simulink model "gm_gmStateSpaceHDL_uz_inverter_3ph"  (R2021b)
settings: Solver=FixedStepDiscrete  StartTime=0.0  StopTime=0.1  FixedStep=Auto  RelTol=1e-3
InitFcn:
  | load('C:\Users\valen\Documents\repos\UZ\ultrazohm_sw_working\ip_cores\uz_inverter_3ph\sschdl\uz_inverter_3ph\stateSpaceParameters.mat');
undefined symbols (not defined in the file or in its folder): udc
libraries: hdlmdlgenlib x140, dspsigops x26, simulink x17, hdlssclib x2
(part 2 of 2)

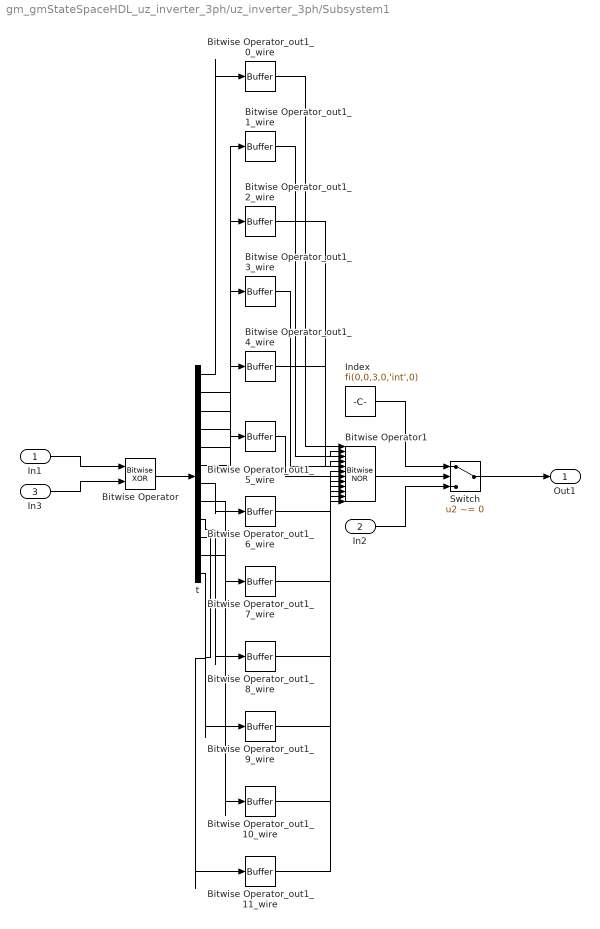
== system gm_gmStateSpaceHDL_uz_inverter_3ph/uz_inverter_3ph/Subsystem1 ==
  In1 : Inport  OutDataTypeStr=boolean  PortDimensions=[12]  SampleTime=1e-08
  In2 : Inport  Port=2  OutDataTypeStr=fixdt(0, 3, 0)  PortDimensions=1  SampleTime=1e-08
  In3 : Inport  Port=3  OutDataTypeStr=boolean  PortDimensions=[12]  SampleTime=1e-08
  Bitwise Operator : simulink/Logic and Bit Operations/Bitwise Operator  logicop=XOR  UseBitMask=off  NumInputPorts=2  BitMask=double(0)  BitMaskRealWorld=Real World Value
  Bitwise Operator1 : simulink/Logic and Bit Operations/Bitwise Operator  logicop=NOR  UseBitMask=off  NumInputPorts=12  BitMask=double(0)  BitMaskRealWorld=Real World Value
  Bitwise Operator_out1_0_wire : hdlmdlgenlib/Buffer
      settings: SourceProductBaseCode=SL
  Bitwise Operator_out1_10_wire : hdlmdlgenlib/Buffer
      settings: SourceProductBaseCode=SL
  Bitwise Operator_out1_11_wire : hdlmdlgenlib/Buffer
      settings: SourceProductBaseCode=SL
  Bitwise Operator_out1_1_wire : hdlmdlgenlib/Buffer
      settings: SourceProductBaseCode=SL
  Bitwise Operator_out1_2_wire : hdlmdlgenlib/Buffer
      settings: SourceProductBaseCode=SL
  Bitwise Operator_out1_3_wire : hdlmdlgenlib/Buffer
      settings: SourceProductBaseCode=SL
  Bitwise Operator_out1_4_wire : hdlmdlgenlib/Buffer
      settings: SourceProductBaseCode=SL
  Bitwise Operator_out1_5_wire : hdlmdlgenlib/Buffer
      settings: SourceProductBaseCode=SL
  Bitwise Operator_out1_6_wire : hdlmdlgenlib/Buffer
      settings: SourceProductBaseCode=SL
  Bitwise Operator_out1_7_wire : hdlmdlgenlib/Buffer
      settings: SourceProductBaseCode=SL
  Bitwise Operator_out1_8_wire : hdlmdlgenlib/Buffer
      settings: SourceProductBaseCode=SL
  Bitwise Operator_out1_9_wire : hdlmdlgenlib/Buffer
      settings: SourceProductBaseCode=SL
  Index : Constant  Value=fi(0,0,3,0,'int',0)  OutDataTypeStr=fixdt(0, 3, 0)  SampleTime=1e-08
  Switch : Switch  Criteria=u2 ~= 0  Threshold=double(0)  OutDataTypeStr=fixdt(0, 3, 0)  SampleTime=1e-08
  t : Demux  Outputs=12
  Out1 : Outport  SampleTime=1e-08  VectorParamsAs1DForOutWhenUnconnected=off
  wires:
  Bitwise Operator/1 -> t/1
  Bitwise Operator1/1 -> Switch/2
  Bitwise Operator_out1_0_wire/1 -> Bitwise Operator1/1
  Bitwise Operator_out1_1_wire/1 -> Bitwise Operator1/2
  Bitwise Operator_out1_2_wire/1 -> Bitwise Operator1/3
  Bitwise Operator_out1_3_wire/1 -> Bitwise Operator1/4
  Bitwise Operator_out1_4_wire/1 -> Bitwise Operator1/5
  Bitwise Operator_out1_5_wire/1 -> Bitwise Operator1/6
  Bitwise Operator_out1_6_wire/1 -> Bitwise Operator1/7
  Bitwise Operator_out1_7_wire/1 -> Bitwise Operator1/8
  Bitwise Operator_out1_8_wire/1 -> Bitwise Operator1/9
  Bitwise Operator_out1_9_wire/1 -> Bitwise Operator1/10
  Bitwise Operator_out1_10_wire/1 -> Bitwise Operator1/11
  Bitwise Operator_out1_11_wire/1 -> Bitwise Operator1/12
  Index/1 -> Switch/1
  Switch/1 -> Out1/1
  t/1 -> Bitwise Operator_out1_0_wire/1
  t/2 -> Bitwise Operator_out1_1_wire/1
  t/3 -> Bitwise Operator_out1_2_wire/1
  t/4 -> Bitwise Operator_out1_3_wire/1
  t/5 -> Bitwise Operator_out1_4_wire/1
  t/6 -> Bitwise Operator_out1_5_wire/1
  t/7 -> Bitwise Operator_out1_6_wire/1
  t/8 -> Bitwise Operator_out1_7_wire/1
  t/9 -> Bitwise Operator_out1_8_wire/1
  t/10 -> Bitwise Operator_out1_9_wire/1
  t/11 -> Bitwise Operator_out1_10_wire/1
  t/12 -> Bitwise Operator_out1_11_wire/1
  In1/1 -> Bitwise Operator/1
  In2/1 -> Switch/3
  In3/1 -> Bitwise Operator/2

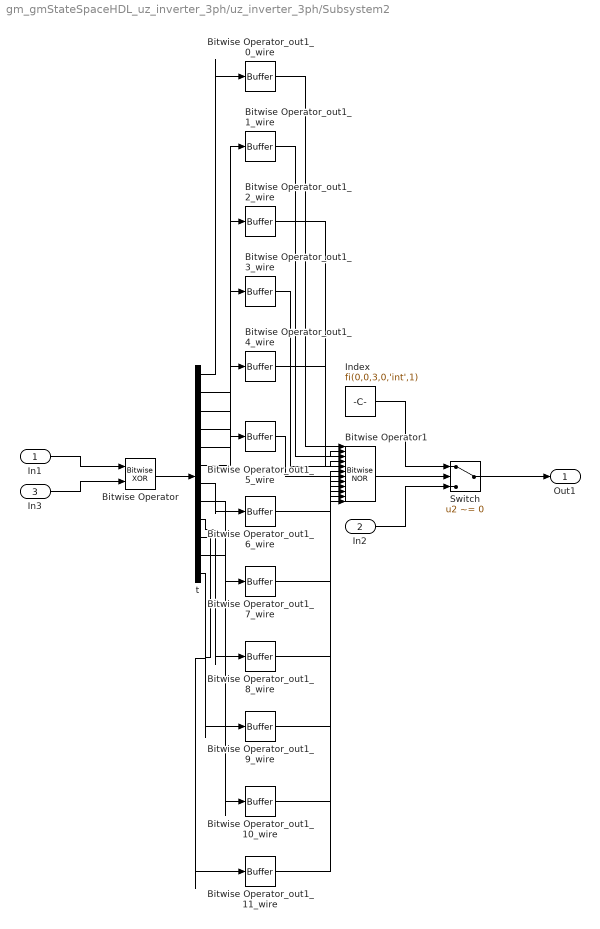
== system gm_gmStateSpaceHDL_uz_inverter_3ph/uz_inverter_3ph/Subsystem2 ==
  In1 : Inport  OutDataTypeStr=boolean  PortDimensions=[12]  SampleTime=1e-08
  In2 : Inport  Port=2  OutDataTypeStr=fixdt(0, 3, 0)  PortDimensions=1  SampleTime=1e-08
  In3 : Inport  Port=3  OutDataTypeStr=boolean  PortDimensions=[12]  SampleTime=1e-08
  Bitwise Operator : simulink/Logic and Bit Operations/Bitwise Operator  logicop=XOR  UseBitMask=off  NumInputPorts=2  BitMask=double(0)  BitMaskRealWorld=Real World Value
  Bitwise Operator1 : simulink/Logic and Bit Operations/Bitwise Operator  logicop=NOR  UseBitMask=off  NumInputPorts=12  BitMask=double(0)  BitMaskRealWorld=Real World Value
  Bitwise Operator_out1_0_wire : hdlmdlgenlib/Buffer
      settings: SourceProductBaseCode=SL
  Bitwise Operator_out1_10_wire : hdlmdlgenlib/Buffer
      settings: SourceProductBaseCode=SL
  Bitwise Operator_out1_11_wire : hdlmdlgenlib/Buffer
      settings: SourceProductBaseCode=SL
  Bitwise Operator_out1_1_wire : hdlmdlgenlib/Buffer
      settings: SourceProductBaseCode=SL
  Bitwise Operator_out1_2_wire : hdlmdlgenlib/Buffer
      settings: SourceProductBaseCode=SL
  Bitwise Operator_out1_3_wire : hdlmdlgenlib/Buffer
      settings: SourceProductBaseCode=SL
  Bitwise Operator_out1_4_wire : hdlmdlgenlib/Buffer
      settings: SourceProductBaseCode=SL
  Bitwise Operator_out1_5_wire : hdlmdlgenlib/Buffer
      settings: SourceProductBaseCode=SL
  Bitwise Operator_out1_6_wire : hdlmdlgenlib/Buffer
      settings: SourceProductBaseCode=SL
  Bitwise Operator_out1_7_wire : hdlmdlgenlib/Buffer
      settings: SourceProductBaseCode=SL
  Bitwise Operator_out1_8_wire : hdlmdlgenlib/Buffer
      settings: SourceProductBaseCode=SL
  Bitwise Operator_out1_9_wire : hdlmdlgenlib/Buffer
      settings: SourceProductBaseCode=SL
  Index : Constant  Value=fi(0,0,3,0,'int',1)  OutDataTypeStr=fixdt(0, 3, 0)  SampleTime=1e-08
  Switch : Switch  Criteria=u2 ~= 0  Threshold=double(0)  OutDataTypeStr=fixdt(0, 3, 0)  SampleTime=1e-08
  t : Demux  Outputs=12
  Out1 : Outport  SampleTime=1e-08  VectorParamsAs1DForOutWhenUnconnected=off
  wires:
  Bitwise Operator/1 -> t/1
  Bitwise Operator1/1 -> Switch/2
  Bitwise Operator_out1_0_wire/1 -> Bitwise Operator1/1
  Bitwise Operator_out1_1_wire/1 -> Bitwise Operator1/2
  Bitwise Operator_out1_2_wire/1 -> Bitwise Operator1/3
  Bitwise Operator_out1_3_wire/1 -> Bitwise Operator1/4
  Bitwise Operator_out1_4_wire/1 -> Bitwise Operator1/5
  Bitwise Operator_out1_5_wire/1 -> Bitwise Operator1/6
  Bitwise Operator_out1_6_wire/1 -> Bitwise Operator1/7
  Bitwise Operator_out1_7_wire/1 -> Bitwise Operator1/8
  Bitwise Operator_out1_8_wire/1 -> Bitwise Operator1/9
  Bitwise Operator_out1_9_wire/1 -> Bitwise Operator1/10
  Bitwise Operator_out1_10_wire/1 -> Bitwise Operator1/11
  Bitwise Operator_out1_11_wire/1 -> Bitwise Operator1/12
  Index/1 -> Switch/1
  Switch/1 -> Out1/1
  t/1 -> Bitwise Operator_out1_0_wire/1
  t/2 -> Bitwise Operator_out1_1_wire/1
  t/3 -> Bitwise Operator_out1_2_wire/1
  t/4 -> Bitwise Operator_out1_3_wire/1
  t/5 -> Bitwise Operator_out1_4_wire/1
  t/6 -> Bitwise Operator_out1_5_wire/1
  t/7 -> Bitwise Operator_out1_6_wire/1
  t/8 -> Bitwise Operator_out1_7_wire/1
  t/9 -> Bitwise Operator_out1_8_wire/1
  t/10 -> Bitwise Operator_out1_9_wire/1
  t/11 -> Bitwise Operator_out1_10_wire/1
  t/12 -> Bitwise Operator_out1_11_wire/1
  In1/1 -> Bitwise Operator/1
  In2/1 -> Switch/3
  In3/1 -> Bitwise Operator/2

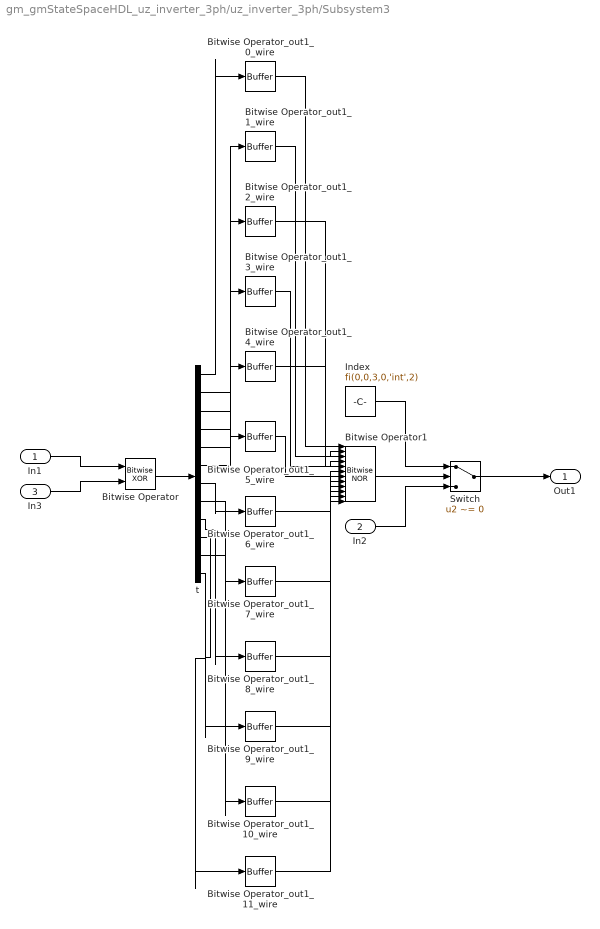
== system gm_gmStateSpaceHDL_uz_inverter_3ph/uz_inverter_3ph/Subsystem3 ==
  In1 : Inport  OutDataTypeStr=boolean  PortDimensions=[12]  SampleTime=1e-08
  In2 : Inport  Port=2  OutDataTypeStr=fixdt(0, 3, 0)  PortDimensions=1  SampleTime=1e-08
  In3 : Inport  Port=3  OutDataTypeStr=boolean  PortDimensions=[12]  SampleTime=1e-08
  Bitwise Operator : simulink/Logic and Bit Operations/Bitwise Operator  logicop=XOR  UseBitMask=off  NumInputPorts=2  BitMask=double(0)  BitMaskRealWorld=Real World Value
  Bitwise Operator1 : simulink/Logic and Bit Operations/Bitwise Operator  logicop=NOR  UseBitMask=off  NumInputPorts=12  BitMask=double(0)  BitMaskRealWorld=Real World Value
  Bitwise Operator_out1_0_wire : hdlmdlgenlib/Buffer
      settings: SourceProductBaseCode=SL
  Bitwise Operator_out1_10_wire : hdlmdlgenlib/Buffer
      settings: SourceProductBaseCode=SL
  Bitwise Operator_out1_11_wire : hdlmdlgenlib/Buffer
      settings: SourceProductBaseCode=SL
  Bitwise Operator_out1_1_wire : hdlmdlgenlib/Buffer
      settings: SourceProductBaseCode=SL
  Bitwise Operator_out1_2_wire : hdlmdlgenlib/Buffer
      settings: SourceProductBaseCode=SL
  Bitwise Operator_out1_3_wire : hdlmdlgenlib/Buffer
      settings: SourceProductBaseCode=SL
  Bitwise Operator_out1_4_wire : hdlmdlgenlib/Buffer
      settings: SourceProductBaseCode=SL
  Bitwise Operator_out1_5_wire : hdlmdlgenlib/Buffer
      settings: SourceProductBaseCode=SL
  Bitwise Operator_out1_6_wire : hdlmdlgenlib/Buffer
      settings: SourceProductBaseCode=SL
  Bitwise Operator_out1_7_wire : hdlmdlgenlib/Buffer
      settings: SourceProductBaseCode=SL
  Bitwise Operator_out1_8_wire : hdlmdlgenlib/Buffer
      settings: SourceProductBaseCode=SL
  Bitwise Operator_out1_9_wire : hdlmdlgenlib/Buffer
      settings: SourceProductBaseCode=SL
  Index : Constant  Value=fi(0,0,3,0,'int',2)  OutDataTypeStr=fixdt(0, 3, 0)  SampleTime=1e-08
  Switch : Switch  Criteria=u2 ~= 0  Threshold=double(0)  OutDataTypeStr=fixdt(0, 3, 0)  SampleTime=1e-08
  t : Demux  Outputs=12
  Out1 : Outport  SampleTime=1e-08  VectorParamsAs1DForOutWhenUnconnected=off
  wires:
  Bitwise Operator/1 -> t/1
  Bitwise Operator1/1 -> Switch/2
  Bitwise Operator_out1_0_wire/1 -> Bitwise Operator1/1
  Bitwise Operator_out1_1_wire/1 -> Bitwise Operator1/2
  Bitwise Operator_out1_2_wire/1 -> Bitwise Operator1/3
  Bitwise Operator_out1_3_wire/1 -> Bitwise Operator1/4
  Bitwise Operator_out1_4_wire/1 -> Bitwise Operator1/5
  Bitwise Operator_out1_5_wire/1 -> Bitwise Operator1/6
  Bitwise Operator_out1_6_wire/1 -> Bitwise Operator1/7
  Bitwise Operator_out1_7_wire/1 -> Bitwise Operator1/8
  Bitwise Operator_out1_8_wire/1 -> Bitwise Operator1/9
  Bitwise Operator_out1_9_wire/1 -> Bitwise Operator1/10
  Bitwise Operator_out1_10_wire/1 -> Bitwise Operator1/11
  Bitwise Operator_out1_11_wire/1 -> Bitwise Operator1/12
  Index/1 -> Switch/1
  Switch/1 -> Out1/1
  t/1 -> Bitwise Operator_out1_0_wire/1
  t/2 -> Bitwise Operator_out1_1_wire/1
  t/3 -> Bitwise Operator_out1_2_wire/1
  t/4 -> Bitwise Operator_out1_3_wire/1
  t/5 -> Bitwise Operator_out1_4_wire/1
  t/6 -> Bitwise Operator_out1_5_wire/1
  t/7 -> Bitwise Operator_out1_6_wire/1
  t/8 -> Bitwise Operator_out1_7_wire/1
  t/9 -> Bitwise Operator_out1_8_wire/1
  t/10 -> Bitwise Operator_out1_9_wire/1
  t/11 -> Bitwise Operator_out1_10_wire/1
  t/12 -> Bitwise Operator_out1_11_wire/1
  In1/1 -> Bitwise Operator/1
  In2/1 -> Switch/3
  In3/1 -> Bitwise Operator/2

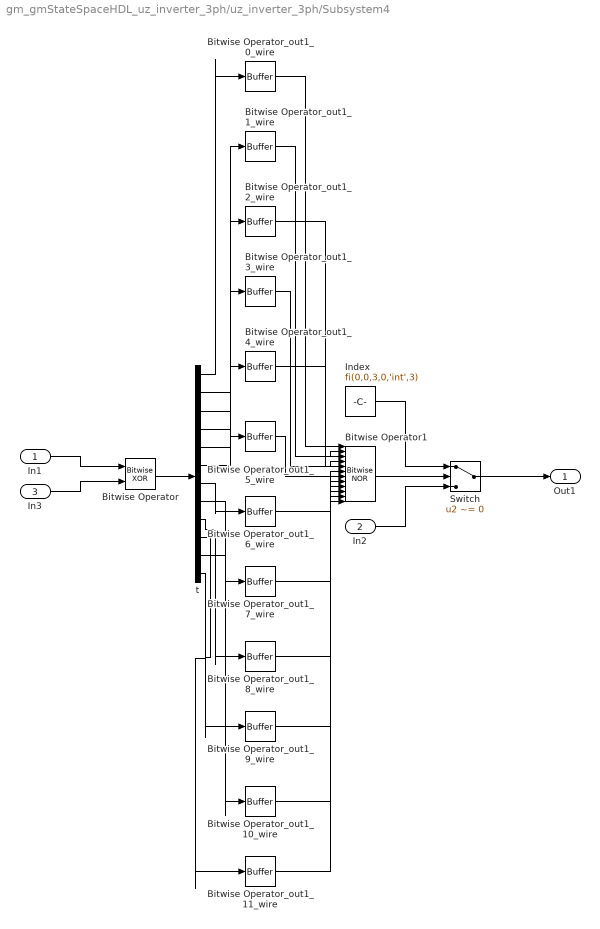
== system gm_gmStateSpaceHDL_uz_inverter_3ph/uz_inverter_3ph/Subsystem4 ==
  In1 : Inport  OutDataTypeStr=boolean  PortDimensions=[12]  SampleTime=1e-08
  In2 : Inport  Port=2  OutDataTypeStr=fixdt(0, 3, 0)  PortDimensions=1  SampleTime=1e-08
  In3 : Inport  Port=3  OutDataTypeStr=boolean  PortDimensions=[12]  SampleTime=1e-08
  Bitwise Operator : simulink/Logic and Bit Operations/Bitwise Operator  logicop=XOR  UseBitMask=off  NumInputPorts=2  BitMask=double(0)  BitMaskRealWorld=Real World Value
  Bitwise Operator1 : simulink/Logic and Bit Operations/Bitwise Operator  logicop=NOR  UseBitMask=off  NumInputPorts=12  BitMask=double(0)  BitMaskRealWorld=Real World Value
  Bitwise Operator_out1_0_wire : hdlmdlgenlib/Buffer
      settings: SourceProductBaseCode=SL
  Bitwise Operator_out1_10_wire : hdlmdlgenlib/Buffer
      settings: SourceProductBaseCode=SL
  Bitwise Operator_out1_11_wire : hdlmdlgenlib/Buffer
      settings: SourceProductBaseCode=SL
  Bitwise Operator_out1_1_wire : hdlmdlgenlib/Buffer
      settings: SourceProductBaseCode=SL
  Bitwise Operator_out1_2_wire : hdlmdlgenlib/Buffer
      settings: SourceProductBaseCode=SL
  Bitwise Operator_out1_3_wire : hdlmdlgenlib/Buffer
      settings: SourceProductBaseCode=SL
  Bitwise Operator_out1_4_wire : hdlmdlgenlib/Buffer
      settings: SourceProductBaseCode=SL
  Bitwise Operator_out1_5_wire : hdlmdlgenlib/Buffer
      settings: SourceProductBaseCode=SL
  Bitwise Operator_out1_6_wire : hdlmdlgenlib/Buffer
      settings: SourceProductBaseCode=SL
  Bitwise Operator_out1_7_wire : hdlmdlgenlib/Buffer
      settings: SourceProductBaseCode=SL
  Bitwise Operator_out1_8_wire : hdlmdlgenlib/Buffer
      settings: SourceProductBaseCode=SL
  Bitwise Operator_out1_9_wire : hdlmdlgenlib/Buffer
      settings: SourceProductBaseCode=SL
  Index : Constant  Value=fi(0,0,3,0,'int',3)  OutDataTypeStr=fixdt(0, 3, 0)  SampleTime=1e-08
  Switch : Switch  Criteria=u2 ~= 0  Threshold=double(0)  OutDataTypeStr=fixdt(0, 3, 0)  SampleTime=1e-08
  t : Demux  Outputs=12
  Out1 : Outport  SampleTime=1e-08  VectorParamsAs1DForOutWhenUnconnected=off
  wires:
  Bitwise Operator/1 -> t/1
  Bitwise Operator1/1 -> Switch/2
  Bitwise Operator_out1_0_wire/1 -> Bitwise Operator1/1
  Bitwise Operator_out1_1_wire/1 -> Bitwise Operator1/2
  Bitwise Operator_out1_2_wire/1 -> Bitwise Operator1/3
  Bitwise Operator_out1_3_wire/1 -> Bitwise Operator1/4
  Bitwise Operator_out1_4_wire/1 -> Bitwise Operator1/5
  Bitwise Operator_out1_5_wire/1 -> Bitwise Operator1/6
  Bitwise Operator_out1_6_wire/1 -> Bitwise Operator1/7
  Bitwise Operator_out1_7_wire/1 -> Bitwise Operator1/8
  Bitwise Operator_out1_8_wire/1 -> Bitwise Operator1/9
  Bitwise Operator_out1_9_wire/1 -> Bitwise Operator1/10
  Bitwise Operator_out1_10_wire/1 -> Bitwise Operator1/11
  Bitwise Operator_out1_11_wire/1 -> Bitwise Operator1/12
  Index/1 -> Switch/1
  Switch/1 -> Out1/1
  t/1 -> Bitwise Operator_out1_0_wire/1
  t/2 -> Bitwise Operator_out1_1_wire/1
  t/3 -> Bitwise Operator_out1_2_wire/1
  t/4 -> Bitwise Operator_out1_3_wire/1
  t/5 -> Bitwise Operator_out1_4_wire/1
  t/6 -> Bitwise Operator_out1_5_wire/1
  t/7 -> Bitwise Operator_out1_6_wire/1
  t/8 -> Bitwise Operator_out1_7_wire/1
  t/9 -> Bitwise Operator_out1_8_wire/1
  t/10 -> Bitwise Operator_out1_9_wire/1
  t/11 -> Bitwise Operator_out1_10_wire/1
  t/12 -> Bitwise Operator_out1_11_wire/1
  In1/1 -> Bitwise Operator/1
  In2/1 -> Switch/3
  In3/1 -> Bitwise Operator/2

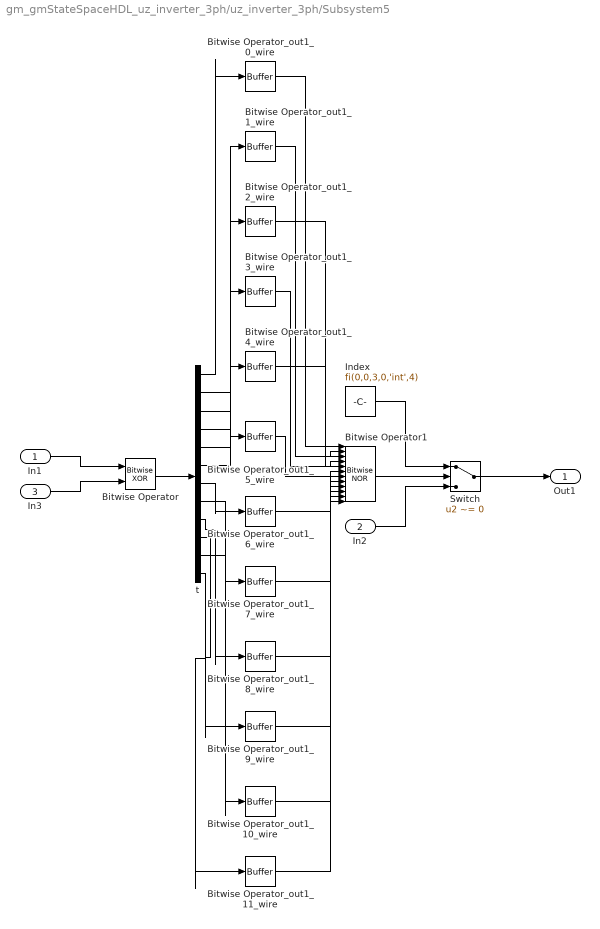
== system gm_gmStateSpaceHDL_uz_inverter_3ph/uz_inverter_3ph/Subsystem5 ==
  In1 : Inport  OutDataTypeStr=boolean  PortDimensions=[12]  SampleTime=1e-08
  In2 : Inport  Port=2  OutDataTypeStr=fixdt(0, 3, 0)  PortDimensions=1  SampleTime=1e-08
  In3 : Inport  Port=3  OutDataTypeStr=boolean  PortDimensions=[12]  SampleTime=1e-08
  Bitwise Operator : simulink/Logic and Bit Operations/Bitwise Operator  logicop=XOR  UseBitMask=off  NumInputPorts=2  BitMask=double(0)  BitMaskRealWorld=Real World Value
  Bitwise Operator1 : simulink/Logic and Bit Operations/Bitwise Operator  logicop=NOR  UseBitMask=off  NumInputPorts=12  BitMask=double(0)  BitMaskRealWorld=Real World Value
  Bitwise Operator_out1_0_wire : hdlmdlgenlib/Buffer
      settings: SourceProductBaseCode=SL
  Bitwise Operator_out1_10_wire : hdlmdlgenlib/Buffer
      settings: SourceProductBaseCode=SL
  Bitwise Operator_out1_11_wire : hdlmdlgenlib/Buffer
      settings: SourceProductBaseCode=SL
  Bitwise Operator_out1_1_wire : hdlmdlgenlib/Buffer
      settings: SourceProductBaseCode=SL
  Bitwise Operator_out1_2_wire : hdlmdlgenlib/Buffer
      settings: SourceProductBaseCode=SL
  Bitwise Operator_out1_3_wire : hdlmdlgenlib/Buffer
      settings: SourceProductBaseCode=SL
  Bitwise Operator_out1_4_wire : hdlmdlgenlib/Buffer
      settings: SourceProductBaseCode=SL
  Bitwise Operator_out1_5_wire : hdlmdlgenlib/Buffer
      settings: SourceProductBaseCode=SL
  Bitwise Operator_out1_6_wire : hdlmdlgenlib/Buffer
      settings: SourceProductBaseCode=SL
  Bitwise Operator_out1_7_wire : hdlmdlgenlib/Buffer
      settings: SourceProductBaseCode=SL
  Bitwise Operator_out1_8_wire : hdlmdlgenlib/Buffer
      settings: SourceProductBaseCode=SL
  Bitwise Operator_out1_9_wire : hdlmdlgenlib/Buffer
      settings: SourceProductBaseCode=SL
  Index : Constant  Value=fi(0,0,3,0,'int',4)  OutDataTypeStr=fixdt(0, 3, 0)  SampleTime=1e-08
  Switch : Switch  Criteria=u2 ~= 0  Threshold=double(0)  OutDataTypeStr=fixdt(0, 3, 0)  SampleTime=1e-08
  t : Demux  Outputs=12
  Out1 : Outport  SampleTime=1e-08  VectorParamsAs1DForOutWhenUnconnected=off
  wires:
  Bitwise Operator/1 -> t/1
  Bitwise Operator1/1 -> Switch/2
  Bitwise Operator_out1_0_wire/1 -> Bitwise Operator1/1
  Bitwise Operator_out1_1_wire/1 -> Bitwise Operator1/2
  Bitwise Operator_out1_2_wire/1 -> Bitwise Operator1/3
  Bitwise Operator_out1_3_wire/1 -> Bitwise Operator1/4
  Bitwise Operator_out1_4_wire/1 -> Bitwise Operator1/5
  Bitwise Operator_out1_5_wire/1 -> Bitwise Operator1/6
  Bitwise Operator_out1_6_wire/1 -> Bitwise Operator1/7
  Bitwise Operator_out1_7_wire/1 -> Bitwise Operator1/8
  Bitwise Operator_out1_8_wire/1 -> Bitwise Operator1/9
  Bitwise Operator_out1_9_wire/1 -> Bitwise Operator1/10
  Bitwise Operator_out1_10_wire/1 -> Bitwise Operator1/11
  Bitwise Operator_out1_11_wire/1 -> Bitwise Operator1/12
  Index/1 -> Switch/1
  Switch/1 -> Out1/1
  t/1 -> Bitwise Operator_out1_0_wire/1
  t/2 -> Bitwise Operator_out1_1_wire/1
  t/3 -> Bitwise Operator_out1_2_wire/1
  t/4 -> Bitwise Operator_out1_3_wire/1
  t/5 -> Bitwise Operator_out1_4_wire/1
  t/6 -> Bitwise Operator_out1_5_wire/1
  t/7 -> Bitwise Operator_out1_6_wire/1
  t/8 -> Bitwise Operator_out1_7_wire/1
  t/9 -> Bitwise Operator_out1_8_wire/1
  t/10 -> Bitwise Operator_out1_9_wire/1
  t/11 -> Bitwise Operator_out1_10_wire/1
  t/12 -> Bitwise Operator_out1_11_wire/1
  In1/1 -> Bitwise Operator/1
  In2/1 -> Switch/3
  In3/1 -> Bitwise Operator/2

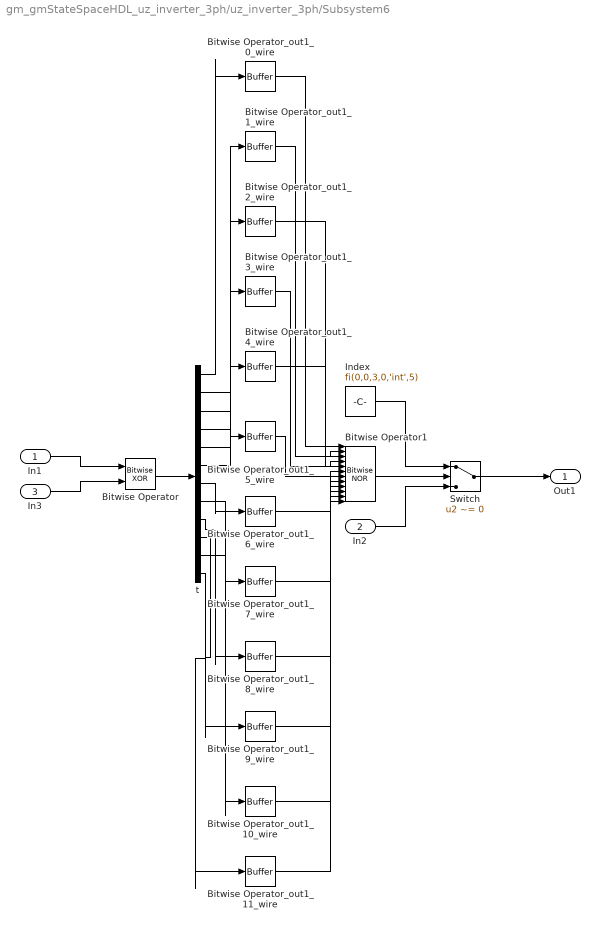
== system gm_gmStateSpaceHDL_uz_inverter_3ph/uz_inverter_3ph/Subsystem6 ==
  In1 : Inport  OutDataTypeStr=boolean  PortDimensions=[12]  SampleTime=1e-08
  In2 : Inport  Port=2  OutDataTypeStr=fixdt(0, 3, 0)  PortDimensions=1  SampleTime=1e-08
  In3 : Inport  Port=3  OutDataTypeStr=boolean  PortDimensions=[12]  SampleTime=1e-08
  Bitwise Operator : simulink/Logic and Bit Operations/Bitwise Operator  logicop=XOR  UseBitMask=off  NumInputPorts=2  BitMask=double(0)  BitMaskRealWorld=Real World Value
  Bitwise Operator1 : simulink/Logic and Bit Operations/Bitwise Operator  logicop=NOR  UseBitMask=off  NumInputPorts=12  BitMask=double(0)  BitMaskRealWorld=Real World Value
  Bitwise Operator_out1_0_wire : hdlmdlgenlib/Buffer
      settings: SourceProductBaseCode=SL
  Bitwise Operator_out1_10_wire : hdlmdlgenlib/Buffer
      settings: SourceProductBaseCode=SL
  Bitwise Operator_out1_11_wire : hdlmdlgenlib/Buffer
      settings: SourceProductBaseCode=SL
  Bitwise Operator_out1_1_wire : hdlmdlgenlib/Buffer
      settings: SourceProductBaseCode=SL
  Bitwise Operator_out1_2_wire : hdlmdlgenlib/Buffer
      settings: SourceProductBaseCode=SL
  Bitwise Operator_out1_3_wire : hdlmdlgenlib/Buffer
      settings: SourceProductBaseCode=SL
  Bitwise Operator_out1_4_wire : hdlmdlgenlib/Buffer
      settings: SourceProductBaseCode=SL
  Bitwise Operator_out1_5_wire : hdlmdlgenlib/Buffer
      settings: SourceProductBaseCode=SL
  Bitwise Operator_out1_6_wire : hdlmdlgenlib/Buffer
      settings: SourceProductBaseCode=SL
  Bitwise Operator_out1_7_wire : hdlmdlgenlib/Buffer
      settings: SourceProductBaseCode=SL
  Bitwise Operator_out1_8_wire : hdlmdlgenlib/Buffer
      settings: SourceProductBaseCode=SL
  Bitwise Operator_out1_9_wire : hdlmdlgenlib/Buffer
      settings: SourceProductBaseCode=SL
  Index : Constant  Value=fi(0,0,3,0,'int',5)  OutDataTypeStr=fixdt(0, 3, 0)  SampleTime=1e-08
  Switch : Switch  Criteria=u2 ~= 0  Threshold=double(0)  OutDataTypeStr=fixdt(0, 3, 0)  SampleTime=1e-08
  t : Demux  Outputs=12
  Out1 : Outport  SampleTime=1e-08  VectorParamsAs1DForOutWhenUnconnected=off
  wires:
  Bitwise Operator/1 -> t/1
  Bitwise Operator1/1 -> Switch/2
  Bitwise Operator_out1_0_wire/1 -> Bitwise Operator1/1
  Bitwise Operator_out1_1_wire/1 -> Bitwise Operator1/2
  Bitwise Operator_out1_2_wire/1 -> Bitwise Operator1/3
  Bitwise Operator_out1_3_wire/1 -> Bitwise Operator1/4
  Bitwise Operator_out1_4_wire/1 -> Bitwise Operator1/5
  Bitwise Operator_out1_5_wire/1 -> Bitwise Operator1/6
  Bitwise Operator_out1_6_wire/1 -> Bitwise Operator1/7
  Bitwise Operator_out1_7_wire/1 -> Bitwise Operator1/8
  Bitwise Operator_out1_8_wire/1 -> Bitwise Operator1/9
  Bitwise Operator_out1_9_wire/1 -> Bitwise Operator1/10
  Bitwise Operator_out1_10_wire/1 -> Bitwise Operator1/11
  Bitwise Operator_out1_11_wire/1 -> Bitwise Operator1/12
  Index/1 -> Switch/1
  Switch/1 -> Out1/1
  t/1 -> Bitwise Operator_out1_0_wire/1
  t/2 -> Bitwise Operator_out1_1_wire/1
  t/3 -> Bitwise Operator_out1_2_wire/1
  t/4 -> Bitwise Operator_out1_3_wire/1
  t/5 -> Bitwise Operator_out1_4_wire/1
  t/6 -> Bitwise Operator_out1_5_wire/1
  t/7 -> Bitwise Operator_out1_6_wire/1
  t/8 -> Bitwise Operator_out1_7_wire/1
  t/9 -> Bitwise Operator_out1_8_wire/1
  t/10 -> Bitwise Operator_out1_9_wire/1
  t/11 -> Bitwise Operator_out1_10_wire/1
  t/12 -> Bitwise Operator_out1_11_wire/1
  In1/1 -> Bitwise Operator/1
  In2/1 -> Switch/3
  In3/1 -> Bitwise Operator/2

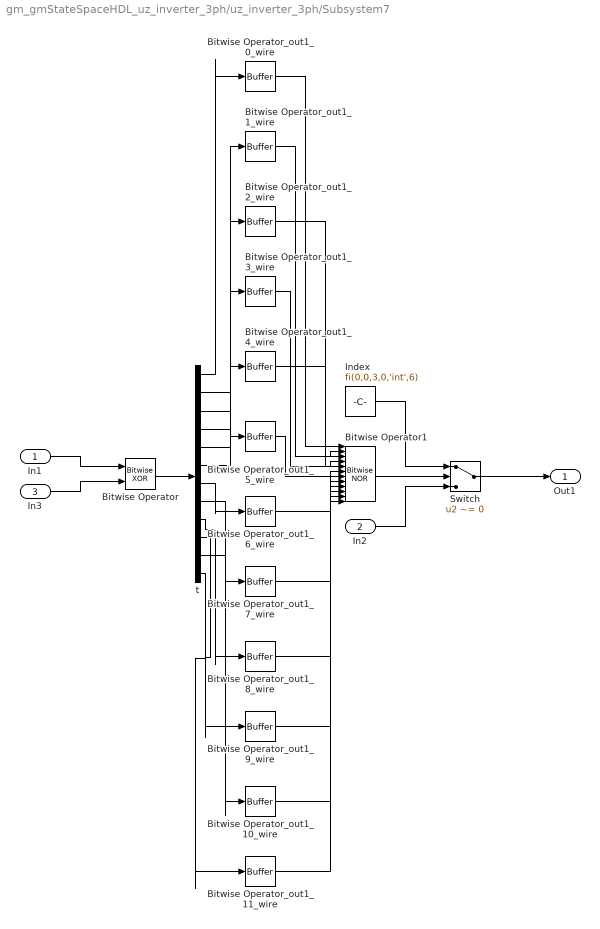
== system gm_gmStateSpaceHDL_uz_inverter_3ph/uz_inverter_3ph/Subsystem7 ==
  In1 : Inport  OutDataTypeStr=boolean  PortDimensions=[12]  SampleTime=1e-08
  In2 : Inport  Port=2  OutDataTypeStr=fixdt(0, 3, 0)  PortDimensions=1  SampleTime=1e-08
  In3 : Inport  Port=3  OutDataTypeStr=boolean  PortDimensions=[12]  SampleTime=1e-08
  Bitwise Operator : simulink/Logic and Bit Operations/Bitwise Operator  logicop=XOR  UseBitMask=off  NumInputPorts=2  BitMask=double(0)  BitMaskRealWorld=Real World Value
  Bitwise Operator1 : simulink/Logic and Bit Operations/Bitwise Operator  logicop=NOR  UseBitMask=off  NumInputPorts=12  BitMask=double(0)  BitMaskRealWorld=Real World Value
  Bitwise Operator_out1_0_wire : hdlmdlgenlib/Buffer
      settings: SourceProductBaseCode=SL
  Bitwise Operator_out1_10_wire : hdlmdlgenlib/Buffer
      settings: SourceProductBaseCode=SL
  Bitwise Operator_out1_11_wire : hdlmdlgenlib/Buffer
      settings: SourceProductBaseCode=SL
  Bitwise Operator_out1_1_wire : hdlmdlgenlib/Buffer
      settings: SourceProductBaseCode=SL
  Bitwise Operator_out1_2_wire : hdlmdlgenlib/Buffer
      settings: SourceProductBaseCode=SL
  Bitwise Operator_out1_3_wire : hdlmdlgenlib/Buffer
      settings: SourceProductBaseCode=SL
  Bitwise Operator_out1_4_wire : hdlmdlgenlib/Buffer
      settings: SourceProductBaseCode=SL
  Bitwise Operator_out1_5_wire : hdlmdlgenlib/Buffer
      settings: SourceProductBaseCode=SL
  Bitwise Operator_out1_6_wire : hdlmdlgenlib/Buffer
      settings: SourceProductBaseCode=SL
  Bitwise Operator_out1_7_wire : hdlmdlgenlib/Buffer
      settings: SourceProductBaseCode=SL
  Bitwise Operator_out1_8_wire : hdlmdlgenlib/Buffer
      settings: SourceProductBaseCode=SL
  Bitwise Operator_out1_9_wire : hdlmdlgenlib/Buffer
      settings: SourceProductBaseCode=SL
  Index : Constant  Value=fi(0,0,3,0,'int',6)  OutDataTypeStr=fixdt(0, 3, 0)  SampleTime=1e-08
  Switch : Switch  Criteria=u2 ~= 0  Threshold=double(0)  OutDataTypeStr=fixdt(0, 3, 0)  SampleTime=1e-08
  t : Demux  Outputs=12
  Out1 : Outport  SampleTime=1e-08  VectorParamsAs1DForOutWhenUnconnected=off
  wires:
  Bitwise Operator/1 -> t/1
  Bitwise Operator1/1 -> Switch/2
  Bitwise Operator_out1_0_wire/1 -> Bitwise Operator1/1
  Bitwise Operator_out1_1_wire/1 -> Bitwise Operator1/2
  Bitwise Operator_out1_2_wire/1 -> Bitwise Operator1/3
  Bitwise Operator_out1_3_wire/1 -> Bitwise Operator1/4
  Bitwise Operator_out1_4_wire/1 -> Bitwise Operator1/5
  Bitwise Operator_out1_5_wire/1 -> Bitwise Operator1/6
  Bitwise Operator_out1_6_wire/1 -> Bitwise Operator1/7
  Bitwise Operator_out1_7_wire/1 -> Bitwise Operator1/8
  Bitwise Operator_out1_8_wire/1 -> Bitwise Operator1/9
  Bitwise Operator_out1_9_wire/1 -> Bitwise Operator1/10
  Bitwise Operator_out1_10_wire/1 -> Bitwise Operator1/11
  Bitwise Operator_out1_11_wire/1 -> Bitwise Operator1/12
  Index/1 -> Switch/1
  Switch/1 -> Out1/1
  t/1 -> Bitwise Operator_out1_0_wire/1
  t/2 -> Bitwise Operator_out1_1_wire/1
  t/3 -> Bitwise Operator_out1_2_wire/1
  t/4 -> Bitwise Operator_out1_3_wire/1
  t/5 -> Bitwise Operator_out1_4_wire/1
  t/6 -> Bitwise Operator_out1_5_wire/1
  t/7 -> Bitwise Operator_out1_6_wire/1
  t/8 -> Bitwise Operator_out1_7_wire/1
  t/9 -> Bitwise Operator_out1_8_wire/1
  t/10 -> Bitwise Operator_out1_9_wire/1
  t/11 -> Bitwise Operator_out1_10_wire/1
  t/12 -> Bitwise Operator_out1_11_wire/1
  In1/1 -> Bitwise Operator/1
  In2/1 -> Switch/3
  In3/1 -> Bitwise Operator/2

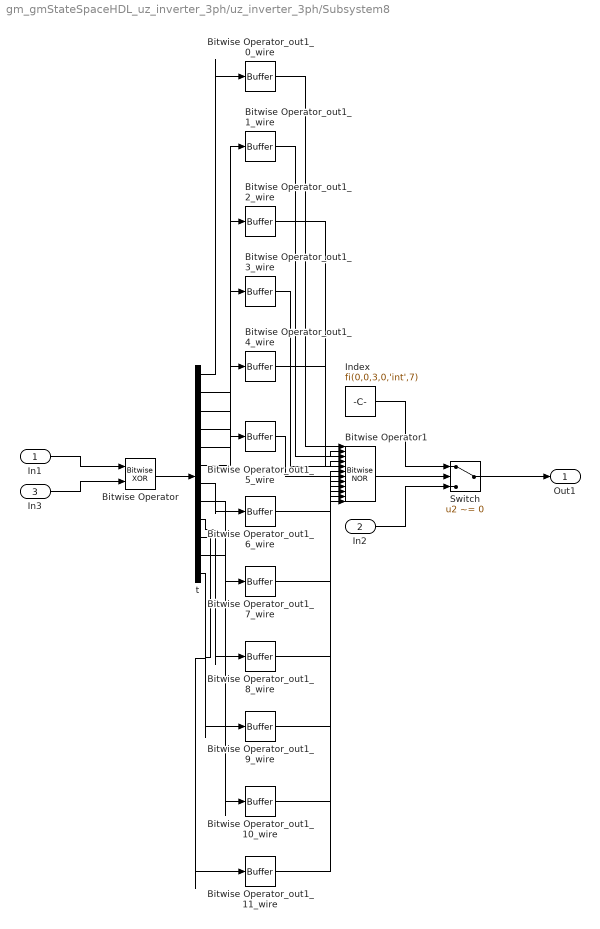
== system gm_gmStateSpaceHDL_uz_inverter_3ph/uz_inverter_3ph/Subsystem8 ==
  In1 : Inport  OutDataTypeStr=boolean  PortDimensions=[12]  SampleTime=1e-08
  In2 : Inport  Port=2  OutDataTypeStr=fixdt(0, 3, 0)  PortDimensions=1  SampleTime=1e-08
  In3 : Inport  Port=3  OutDataTypeStr=boolean  PortDimensions=[12]  SampleTime=1e-08
  Bitwise Operator : simulink/Logic and Bit Operations/Bitwise Operator  logicop=XOR  UseBitMask=off  NumInputPorts=2  BitMask=double(0)  BitMaskRealWorld=Real World Value
  Bitwise Operator1 : simulink/Logic and Bit Operations/Bitwise Operator  logicop=NOR  UseBitMask=off  NumInputPorts=12  BitMask=double(0)  BitMaskRealWorld=Real World Value
  Bitwise Operator_out1_0_wire : hdlmdlgenlib/Buffer
      settings: SourceProductBaseCode=SL
  Bitwise Operator_out1_10_wire : hdlmdlgenlib/Buffer
      settings: SourceProductBaseCode=SL
  Bitwise Operator_out1_11_wire : hdlmdlgenlib/Buffer
      settings: SourceProductBaseCode=SL
  Bitwise Operator_out1_1_wire : hdlmdlgenlib/Buffer
      settings: SourceProductBaseCode=SL
  Bitwise Operator_out1_2_wire : hdlmdlgenlib/Buffer
      settings: SourceProductBaseCode=SL
  Bitwise Operator_out1_3_wire : hdlmdlgenlib/Buffer
      settings: SourceProductBaseCode=SL
  Bitwise Operator_out1_4_wire : hdlmdlgenlib/Buffer
      settings: SourceProductBaseCode=SL
  Bitwise Operator_out1_5_wire : hdlmdlgenlib/Buffer
      settings: SourceProductBaseCode=SL
  Bitwise Operator_out1_6_wire : hdlmdlgenlib/Buffer
      settings: SourceProductBaseCode=SL
  Bitwise Operator_out1_7_wire : hdlmdlgenlib/Buffer
      settings: SourceProductBaseCode=SL
  Bitwise Operator_out1_8_wire : hdlmdlgenlib/Buffer
      settings: SourceProductBaseCode=SL
  Bitwise Operator_out1_9_wire : hdlmdlgenlib/Buffer
      settings: SourceProductBaseCode=SL
  Index : Constant  Value=fi(0,0,3,0,'int',7)  OutDataTypeStr=fixdt(0, 3, 0)  SampleTime=1e-08
  Switch : Switch  Criteria=u2 ~= 0  Threshold=double(0)  OutDataTypeStr=fixdt(0, 3, 0)  SampleTime=1e-08
  t : Demux  Outputs=12
  Out1 : Outport  SampleTime=1e-08  VectorParamsAs1DForOutWhenUnconnected=off
  wires:
  Bitwise Operator/1 -> t/1
  Bitwise Operator1/1 -> Switch/2
  Bitwise Operator_out1_0_wire/1 -> Bitwise Operator1/1
  Bitwise Operator_out1_1_wire/1 -> Bitwise Operator1/2
  Bitwise Operator_out1_2_wire/1 -> Bitwise Operator1/3
  Bitwise Operator_out1_3_wire/1 -> Bitwise Operator1/4
  Bitwise Operator_out1_4_wire/1 -> Bitwise Operator1/5
  Bitwise Operator_out1_5_wire/1 -> Bitwise Operator1/6
  Bitwise Operator_out1_6_wire/1 -> Bitwise Operator1/7
  Bitwise Operator_out1_7_wire/1 -> Bitwise Operator1/8
  Bitwise Operator_out1_8_wire/1 -> Bitwise Operator1/9
  Bitwise Operator_out1_9_wire/1 -> Bitwise Operator1/10
  Bitwise Operator_out1_10_wire/1 -> Bitwise Operator1/11
  Bitwise Operator_out1_11_wire/1 -> Bitwise Operator1/12
  Index/1 -> Switch/1
  Switch/1 -> Out1/1
  t/1 -> Bitwise Operator_out1_0_wire/1
  t/2 -> Bitwise Operator_out1_1_wire/1
  t/3 -> Bitwise Operator_out1_2_wire/1
  t/4 -> Bitwise Operator_out1_3_wire/1
  t/5 -> Bitwise Operator_out1_4_wire/1
  t/6 -> Bitwise Operator_out1_5_wire/1
  t/7 -> Bitwise Operator_out1_6_wire/1
  t/8 -> Bitwise Operator_out1_7_wire/1
  t/9 -> Bitwise Operator_out1_8_wire/1
  t/10 -> Bitwise Operator_out1_9_wire/1
  t/11 -> Bitwise Operator_out1_10_wire/1
  t/12 -> Bitwise Operator_out1_11_wire/1
  In1/1 -> Bitwise Operator/1
  In2/1 -> Switch/3
  In3/1 -> Bitwise Operator/2

== system gm_gmStateSpaceHDL_uz_inverter_3ph/uz_inverter_3ph/adder ==
  In1 : Inport
  In2 : Inport  Port=2
  adder : Sum  OutDataTypeStr=single  SampleTime=1e-08
  adder_pd1 : Delay  DelayLength=6
  Out1 : Outport
  wires:
  In1/1 -> adder/1
  In2/1 -> adder/2
  adder/1 -> adder_pd1/1
  adder_pd1/1 -> Out1/1

== system gm_gmStateSpaceHDL_uz_inverter_3ph/uz_inverter_3ph/adder1 ==
  In1 : Inport
  In2 : Inport  Port=2
  adder1 : Sum  OutDataTypeStr=single  SampleTime=1e-08
  adder1_pd1 : Delay  DelayLength=6
  Out1 : Outport
  wires:
  In1/1 -> adder1/1
  In2/1 -> adder1/2
  adder1/1 -> adder1_pd1/1
  adder1_pd1/1 -> Out1/1

== system gm_gmStateSpaceHDL_uz_inverter_3ph/uz_inverter_3ph/adder2 ==
  In1 : Inport
  In2 : Inport  Port=2
  adder2 : Sum  OutDataTypeStr=single  SampleTime=1e-08
  adder2_pd1 : Delay  DelayLength=6
  Out1 : Outport
  wires:
  In1/1 -> adder2/1
  In2/1 -> adder2/2
  adder2/1 -> adder2_pd1/1
  adder2_pd1/1 -> Out1/1

== system gm_gmStateSpaceHDL_uz_inverter_3ph/uz_inverter_3ph/adder3 ==
  In1 : Inport
  In2 : Inport  Port=2
  adder3 : Sum  OutDataTypeStr=single  SampleTime=1e-08
  adder3_pd1 : Delay  DelayLength=6
  Out1 : Outport
  wires:
  In1/1 -> adder3/1
  In2/1 -> adder3/2
  adder3/1 -> adder3_pd1/1
  adder3_pd1/1 -> Out1/1

== system gm_gmStateSpaceHDL_uz_inverter_3ph/uz_inverter_3ph/adder4 ==
  In1 : Inport
  In2 : Inport  Port=2
  adder4 : Sum  OutDataTypeStr=single  SampleTime=1e-08
  adder4_pd1 : Delay  DelayLength=6
  Out1 : Outport
  wires:
  In1/1 -> adder4/1
  In2/1 -> adder4/2
  adder4/1 -> adder4_pd1/1
  adder4_pd1/1 -> Out1/1

== system gm_gmStateSpaceHDL_uz_inverter_3ph/uz_inverter_3ph/adder5 ==
  In1 : Inport
  In2 : Inport  Port=2
  adder5 : Sum  OutDataTypeStr=single  SampleTime=1e-08
  adder5_pd1 : Delay  DelayLength=6
  Out1 : Outport
  wires:
  In1/1 -> adder5/1
  In2/1 -> adder5/2
  adder5/1 -> adder5_pd1/1
  adder5_pd1/1 -> Out1/1

== system gm_gmStateSpaceHDL_uz_inverter_3ph/uz_inverter_3ph/compare_relop ==
  In1 : Inport
  In2 : Inport  Port=2
  compare_relop : RelationalOperator  Operator=>  OutDataTypeStr=boolean  SampleTime=1e-08  RndMeth=Nearest  InputSameDT=on
  compare_relop_pd1 : Delay  DelayLength=1
  Out1 : Outport
  wires:
  In1/1 -> compare_relop/1
  In2/1 -> compare_relop/2
  compare_relop/1 -> compare_relop_pd1/1
  compare_relop_pd1/1 -> Out1/1

== system gm_gmStateSpaceHDL_uz_inverter_3ph/uz_inverter_3ph/compare_relop1 ==
  In1 : Inport
  In2 : Inport  Port=2
  compare_relop1 : RelationalOperator  Operator=>  OutDataTypeStr=boolean  SampleTime=1e-08  RndMeth=Nearest  InputSameDT=on
  compare_relop1_pd1 : Delay  DelayLength=1
  Out1 : Outport
  wires:
  In1/1 -> compare_relop1/1
  In2/1 -> compare_relop1/2
  compare_relop1/1 -> compare_relop1_pd1/1
  compare_relop1_pd1/1 -> Out1/1

== system gm_gmStateSpaceHDL_uz_inverter_3ph/uz_inverter_3ph/compare_relop10 ==
  In1 : Inport
  In2 : Inport  Port=2
  compare_relop10 : RelationalOperator  Operator=>  OutDataTypeStr=boolean  SampleTime=1e-08  RndMeth=Nearest  InputSameDT=on
  compare_relop10_pd1 : Delay  DelayLength=1
  Out1 : Outport
  wires:
  In1/1 -> compare_relop10/1
  In2/1 -> compare_relop10/2
  compare_relop10/1 -> compare_relop10_pd1/1
  compare_relop10_pd1/1 -> Out1/1

== system gm_gmStateSpaceHDL_uz_inverter_3ph/uz_inverter_3ph/compare_relop11 ==
  In1 : Inport
  In2 : Inport  Port=2
  compare_relop11 : RelationalOperator  Operator=>  OutDataTypeStr=boolean  SampleTime=1e-08  RndMeth=Nearest  InputSameDT=on
  compare_relop11_pd1 : Delay  DelayLength=1
  Out1 : Outport
  wires:
  In1/1 -> compare_relop11/1
  In2/1 -> compare_relop11/2
  compare_relop11/1 -> compare_relop11_pd1/1
  compare_relop11_pd1/1 -> Out1/1

== system gm_gmStateSpaceHDL_uz_inverter_3ph/uz_inverter_3ph/compare_relop2 ==
  In1 : Inport
  In2 : Inport  Port=2
  compare_relop2 : RelationalOperator  Operator=>  OutDataTypeStr=boolean  SampleTime=1e-08  RndMeth=Nearest  InputSameDT=on
  compare_relop2_pd1 : Delay  DelayLength=1
  Out1 : Outport
  wires:
  In1/1 -> compare_relop2/1
  In2/1 -> compare_relop2/2
  compare_relop2/1 -> compare_relop2_pd1/1
  compare_relop2_pd1/1 -> Out1/1

== system gm_gmStateSpaceHDL_uz_inverter_3ph/uz_inverter_3ph/compare_relop3 ==
  In1 : Inport
  In2 : Inport  Port=2
  compare_relop3 : RelationalOperator  Operator=>  OutDataTypeStr=boolean  SampleTime=1e-08  RndMeth=Nearest  InputSameDT=on
  compare_relop3_pd1 : Delay  DelayLength=1
  Out1 : Outport
  wires:
  In1/1 -> compare_relop3/1
  In2/1 -> compare_relop3/2
  compare_relop3/1 -> compare_relop3_pd1/1
  compare_relop3_pd1/1 -> Out1/1

== system gm_gmStateSpaceHDL_uz_inverter_3ph/uz_inverter_3ph/compare_relop4 ==
  In1 : Inport
  In2 : Inport  Port=2
  compare_relop4 : RelationalOperator  Operator=>  OutDataTypeStr=boolean  SampleTime=1e-08  RndMeth=Nearest  InputSameDT=on
  compare_relop4_pd1 : Delay  DelayLength=1
  Out1 : Outport
  wires:
  In1/1 -> compare_relop4/1
  In2/1 -> compare_relop4/2
  compare_relop4/1 -> compare_relop4_pd1/1
  compare_relop4_pd1/1 -> Out1/1

== system gm_gmStateSpaceHDL_uz_inverter_3ph/uz_inverter_3ph/compare_relop5 ==
  In1 : Inport
  In2 : Inport  Port=2
  compare_relop5 : RelationalOperator  Operator=>  OutDataTypeStr=boolean  SampleTime=1e-08  RndMeth=Nearest  InputSameDT=on
  compare_relop5_pd1 : Delay  DelayLength=1
  Out1 : Outport
  wires:
  In1/1 -> compare_relop5/1
  In2/1 -> compare_relop5/2
  compare_relop5/1 -> compare_relop5_pd1/1
  compare_relop5_pd1/1 -> Out1/1

== system gm_gmStateSpaceHDL_uz_inverter_3ph/uz_inverter_3ph/compare_relop6 ==
  In1 : Inport
  In2 : Inport  Port=2
  compare_relop6 : RelationalOperator  Operator=>  OutDataTypeStr=boolean  SampleTime=1e-08  RndMeth=Nearest  InputSameDT=on
  compare_relop6_pd1 : Delay  DelayLength=1
  Out1 : Outport
  wires:
  In1/1 -> compare_relop6/1
  In2/1 -> compare_relop6/2
  compare_relop6/1 -> compare_relop6_pd1/1
  compare_relop6_pd1/1 -> Out1/1

== system gm_gmStateSpaceHDL_uz_inverter_3ph/uz_inverter_3ph/compare_relop7 ==
  In1 : Inport
  In2 : Inport  Port=2
  compare_relop7 : RelationalOperator  Operator=>  OutDataTypeStr=boolean  SampleTime=1e-08  RndMeth=Nearest  InputSameDT=on
  compare_relop7_pd1 : Delay  DelayLength=1
  Out1 : Outport
  wires:
  In1/1 -> compare_relop7/1
  In2/1 -> compare_relop7/2
  compare_relop7/1 -> compare_relop7_pd1/1
  compare_relop7_pd1/1 -> Out1/1

== system gm_gmStateSpaceHDL_uz_inverter_3ph/uz_inverter_3ph/compare_relop8 ==
  In1 : Inport
  In2 : Inport  Port=2
  compare_relop8 : RelationalOperator  Operator=>  OutDataTypeStr=boolean  SampleTime=1e-08  RndMeth=Nearest  InputSameDT=on
  compare_relop8_pd1 : Delay  DelayLength=1
  Out1 : Outport
  wires:
  In1/1 -> compare_relop8/1
  In2/1 -> compare_relop8/2
  compare_relop8/1 -> compare_relop8_pd1/1
  compare_relop8_pd1/1 -> Out1/1

== system gm_gmStateSpaceHDL_uz_inverter_3ph/uz_inverter_3ph/compare_relop9 ==
  In1 : Inport
  In2 : Inport  Port=2
  compare_relop9 : RelationalOperator  Operator=>  OutDataTypeStr=boolean  SampleTime=1e-08  RndMeth=Nearest  InputSameDT=on
  compare_relop9_pd1 : Delay  DelayLength=1
  Out1 : Outport
  wires:
  In1/1 -> compare_relop9/1
  In2/1 -> compare_relop9/2
  compare_relop9/1 -> compare_relop9_pd1/1
  compare_relop9_pd1/1 -> Out1/1

== system gm_gmStateSpaceHDL_uz_inverter_3ph/uz_inverter_3ph/gain_unaryminus ==
  In1 : Inport
  gain_unaryminus : UnaryMinus  SampleTime=1e-08
  Out1 : Outport
  wires:
  In1/1 -> gain_unaryminus/1
  gain_unaryminus/1 -> Out1/1

== system gm_gmStateSpaceHDL_uz_inverter_3ph/uz_inverter_3ph/gain_unaryminus1 ==
  In1 : Inport
  gain_unaryminus1 : UnaryMinus  SampleTime=1e-08
  Out1 : Outport
  wires:
  In1/1 -> gain_unaryminus1/1
  gain_unaryminus1/1 -> Out1/1

== system gm_gmStateSpaceHDL_uz_inverter_3ph/uz_inverter_3ph/gain_unaryminus2 ==
  In1 : Inport
  gain_unaryminus2 : UnaryMinus  SampleTime=1e-08
  Out1 : Outport
  wires:
  In1/1 -> gain_unaryminus2/1
  gain_unaryminus2/1 -> Out1/1

== system gm_gmStateSpaceHDL_uz_inverter_3ph/uz_inverter_3ph/gain_unaryminus3 ==
  In1 : Inport
  gain_unaryminus3 : UnaryMinus  SampleTime=1e-08
  Out1 : Outport
  wires:
  In1/1 -> gain_unaryminus3/1
  gain_unaryminus3/1 -> Out1/1

== system gm_gmStateSpaceHDL_uz_inverter_3ph/uz_inverter_3ph/gain_unaryminus4 ==
  In1 : Inport
  gain_unaryminus4 : UnaryMinus  SampleTime=1e-08
  Out1 : Outport
  wires:
  In1/1 -> gain_unaryminus4/1
  gain_unaryminus4/1 -> Out1/1

== system gm_gmStateSpaceHDL_uz_inverter_3ph/uz_inverter_3ph/gain_unaryminus5 ==
  In1 : Inport
  gain_unaryminus5 : UnaryMinus  SampleTime=1e-08
  Out1 : Outport
  wires:
  In1/1 -> gain_unaryminus5/1
  gain_unaryminus5/1 -> Out1/1

== system gm_gmStateSpaceHDL_uz_inverter_3ph/uz_inverter_3ph/gain_unaryminus6 ==
  In1 : Inport
  gain_unaryminus6 : UnaryMinus  SampleTime=1e-08
  Out1 : Outport
  wires:
  In1/1 -> gain_unaryminus6/1
  gain_unaryminus6/1 -> Out1/1

== system gm_gmStateSpaceHDL_uz_inverter_3ph/uz_inverter_3ph/gain_unaryminus7 ==
  In1 : Inport
  gain_unaryminus7 : UnaryMinus  SampleTime=1e-08
  Out1 : Outport
  wires:
  In1/1 -> gain_unaryminus7/1
  gain_unaryminus7/1 -> Out1/1

== system gm_gmStateSpaceHDL_uz_inverter_3ph/uz_inverter_3ph/gain_unaryminus8 ==
  In1 : Inport
  gain_unaryminus8 : UnaryMinus  SampleTime=1e-08
  Out1 : Outport
  wires:
  In1/1 -> gain_unaryminus8/1
  gain_unaryminus8/1 -> Out1/1
